simulink model "SMDFR"  (R2024b)
settings: Solver=ode15s  StartTime=1  StopTime=1200  FixedStep=0.01  RelTol=1e-3
model workspace (MAT data in the model file):
  ACS_lambda = 0.000161129786201
  A_cucl = 134.446
  A_cucl2 = 134.446
  A_cuocl = 213.991
  A_d = 217.647058824
  A_fw = [13.6 90 13.6]
  A_h = 217.647058824
  A_h2 = 217.647058824
  A_h20 = 18.015
  A_hcl = 36.458
  A_o = 32
  A_sg = 370
  A_wc = [10.9 103 10.9]
  C_c = 140.2
  C_cucl = 0.71
  C_cuocl = 1
  C_dst = 1996000
  C_h20 = 4.48
  C_hcl = 0.8
  C_hst = 1996000
  C_i0 = [429000000000000; 4.15e+15; 3.83e+15; 1.16e+16; 5.7e+15; 1.53e+15]
  C_o = 0.918
  Ce_i0 = [701000000000000; 5.88e+15; 3.36e+15; 5.09e+15; 820000000000000; 39600000000000]
  Cr = 0.00113148387097
  Cr_m = 8.769
  Cr_m_red = 4.3845
  Cr_red = 0.000565741935484
  D = 0.16
  DPB_lambda = 0.01
  EPB_lambda = 0.01
  E_d = 5
  E_e = 5
  E_h = 5
  E_hte = 5
  G_cucl = 44.778
  G_cucl2 = 44.778
  G_cuocl = 35.6355
  G_h2 = 32
  G_h20 = 10
  G_h20i = 10
  G_h20o = 7
  G_hcl = 12.1426
  G_o = 2.66
  G_s = 27000
  H_valve = 1
  Heat = [18744000 5970000 16956000]
  IPB_lambda = 0.01
  K_d = 500
  K_h = 500
  L = 6
  LOCA1 = 0
  LOCA2 = 0
  LOCA3 = 0
  LOCA4 = 0
  LOCA_p = 0.000161129786201
  LOCA_time = 300
  LOCA_times = [408 453 64 457 317 49 140 274 479 483 79 486 ... (4000 elements, 1000x4)]
  LOPC = 0
  LOPC_p = 0.1
  LOPC_times = [214 478 363 291 271 353 3 392 464 5 413 384 ... (1000 elements, 1000x1)]
  L_ACS = 0.01
  Lambda = 1.05e-06
  M_c = [219.9 7705 219.9]
  M_cucl0 = 44.778
  M_cucl20 = 44.778
  M_f = [307.7 1164 307.7]
  M_h20 = 8
  M_hcl0 = 12.1426
  M_w = [39.3 311 39.3]
  N = 1000
  N_0 = 15000000000000
  Nodes = 3
  P_0 = 100000000
  P_decomposition = 160
  P_hydro = 167
  Pb_acs : object (value not decoded)
  Pb_pipes : object (value not decoded)
  Pi_0 = [0.158 0.6899 0.152]
  Power_lambda = 0.01
  RPB_lambda = 0.01
  T_fw = 300
  T_hpi = 100
  T_st = 900
  Tbar_c0 = 1060
  Tbar_f0 = 1288
  Tc_in = 973
  Tin_c = 973
  Tin_f = 1300
  Tout_c = 1100
  Tout_f = 1300
  V_c = 160
  V_d = 160
  V_dst = 100
  V_h = 160
  V_h2 = 160
  V_hst = 100
  V_s = 100
  V_sg = 100
  age = 0
  ages = [0 50]
  alfa_c = -8.28e-06
  alfa_f = -0.000208
  alpha = 0.9926
  alpha_1 = 1
  alpha_2 = 1
  alpha_3 = 1
  alpha_4 = 1
  beta = 0.00302
  beta_i = [7.91e-05 0.000703 0.000504 0.00117 0.000457 0.00011]
  c_pc = [140.2 140.2 140.2]
  c_pf = [400 400 400]
  c_pw = [690 690 690]
  coolpipes = [2166 2166 0]
  d_c = 10187.40024
  d_dst = 3.14
  d_hst = 3.14
  d_st = 6.123
  diesel_lambda = 0.01
  eta = 0.4
  fail_threshold = 1244
  file = 'SMDFR_Parameters'
  fuelpipes = 1027
  h_dpo = 6801000
  h_fw = [6546 4305.1 7629.5]
  h_fw_st = 4386450
  h_hpo = 7159680
  h_in = 7000
  h_out = 1000
  h_st_in = 4386450
  h_wc = [27405.4 13833.4 32177.3]
  i = 1
  j = 1
  k_d = 2.7187
  k_e = 2.7187
  k_h = 0.005
  k_hte = 2.7187
  k_sg = 500
  lambda_c = 0.184
  lambda_e = 0.1
  lambda_i = [0.0127 0.03 0.11 0.319 1.18 7.02]
  leakage = 6.5
  mdot_c = [5550.5 5550.5 5550.5]
  mdot_c_value = 5550.5
  mdot_f = [327.7 327.7 327.7]
  mdot_f_value = 327.7
  model = 'SMDFR'
  mu = 50.9722799688
  mu_f = -20.9722799688
  mu_o = 30
  n = 0.45
  nsim = 1
  p_h20 = 40
  phi_tot = 3.61e+21
  rho = 7750
  rho_0 = 0.00111
  rhoex_value = 0
  sigma = 625
  sigma_c = 5
  sigma_f = 5.83095189485
  sigma_o = 3
  step = 0.1
  t = 0.008
  tau_c = 5.43
  tau_e = 10
  tsim = 500
  v_rec = 4.16e-09
values from neighbouring files (symbols this model uses):
  ACS1_flow = 25    [Simulation_model.m]
  ACS1_response_time = randi(t_max_r_ACS-t_min_r_ACS)+t_min_r_ACS    [Failure_model.m]    (also in Failure_model_outputs.mat = 38)
  ACS2_flow = 25    [Simulation_model.m]
  ACS2_response_time = randi(t_max_r_ACS-t_min_r_ACS)+t_min_r_ACS    [Failure_model.m]    (also in Failure_model_outputs.mat = 82)
  ACS3_flow = 25    [Simulation_model.m]
  ACS3_response_time = randi(t_max_r_ACS-t_min_r_ACS)+t_min_r_ACS    [Failure_model.m]    (also in Failure_model_outputs.mat = 78)
  ACS4_flow = 25    [Simulation_model.m]
  ACS4_response_time = randi(t_max_r_ACS-t_min_r_ACS)+t_min_r_ACS    [Failure_model.m]    (also in Failure_model_outputs.mat = 42)
  ACS_1 = 1065    [Failure_model_outputs.mat]    (also in Failure_sim.m = 1200; Failure_sim_HTE_model.m = 1200)
  ACS_2 = 740    [Failure_model_outputs.mat]    (also in Failure_sim.m = 1200; Failure_sim_HTE_model.m = 1200)
  ACS_3 = 745    [Failure_model_outputs.mat]    (also in Failure_sim.m = 1200; Failure_sim_HTE_model.m = 1200)
  ACS_4 = 1055    [Failure_model_outputs.mat]    (also in Failure_sim.m = 1200; Failure_sim_HTE_model.m = 1200)
  All_Outputs = 0    [Simulation_model.m]
  EDG1_response_time = randi(t_max_r_EDG-t_min_r_EDG)+t_min_r_EDG    [Failure_model.m]    (also in Failure_model_outputs.mat = 40)
  EDG2_response_time = randi(t_max_r_EDG-t_min_r_EDG)+t_min_r_EDG    [Failure_model.m]    (also in Failure_model_outputs.mat = 125)
  EDG_1 = 203    [Failure_model_outputs.mat]
  EDG_2 = 296    [Failure_model_outputs.mat]
  LOCA1_time = 1200    [Failure_model_outputs.mat]    (also in Failure_sim.m; Failure_sim_HTE_model.m)
  LOCA2_time = 2    [Failure_model_outputs.mat]    (also in Failure_sim.m = 1200; Failure_sim_HTE_model.m = 1200)
  LOCA3_time = 1200    [Failure_model_outputs.mat]    (also in Failure_sim.m; Failure_sim_HTE_model.m)
  LOCA4_time = 4    [Failure_model_outputs.mat]    (also in Failure_sim.m = 1200; Failure_sim_HTE_model.m = 1200)
  MSLB1 = 1200    [Failure_model_outputs.mat]    (also in Failure_sim.m = fix(randsample(x_loca, 1, true, lognorm_pdf)); Failure_sim_HTE_model.m = fix(randsample(x_loca, 1, true, lognorm_pdf)))
  MSLB2 = 1200    [Failure_model_outputs.mat]    (also in Failure_sim.m = fix(randsample(x_loca, 1, true, lognorm_pdf)); Failure_sim_HTE_model.m = fix(randsample(x_loca, 1, true, lognorm_pdf)))
  MSLB3 = 1200    [Failure_model_outputs.mat]    (also in Failure_sim.m = fix(randsample(x_loca, 1, true, lognorm_pdf)); Failure_sim_HTE_model.m = fix(randsample(x_loca, 1, true, lognorm_pdf)))
  MSLB4 = 1200    [Failure_model_outputs.mat]    (also in Failure_sim.m = fix(randsample(x_loca, 1, true, lognorm_pdf)); Failure_sim_HTE_model.m = fix(randsample(x_loca, 1, true, lognorm_pdf)))
  PDP11 = 1200    [Failure_model_outputs.mat]    (also in Failure_sim.m = t_min_EDG+randi(t_max_EDG-t_min_EDG); Failure_sim_HTE_model.m = t_min_EDG+randi(t_max_EDG-t_min_EDG))
  PDP11_response_time = randi(t_max_r_EDG-t_min_r_EDG)+t_min_r_EDG    [Failure_model.m]    (also in Failure_model_outputs.mat = 78)
  PDP12 = 1200    [Failure_model_outputs.mat]    (also in Failure_sim.m = t_min_EDG+randi(t_max_EDG-t_min_EDG); Failure_sim_HTE_model.m = t_min_EDG+randi(t_max_EDG-t_min_EDG))
  PDP12_response_time = randi(t_max_r_EDG-t_min_r_EDG)+t_min_r_EDG    [Failure_model.m]    (also in Failure_model_outputs.mat = 170)
  PDP21 = 1200    [Failure_model_outputs.mat]    (also in Failure_sim.m = t_min_EDG+randi(t_max_EDG-t_min_EDG); Failure_sim_HTE_model.m = t_min_EDG+randi(t_max_EDG-t_min_EDG))
  PDP21_response_time = randi(t_max_r_EDG-t_min_r_EDG)+t_min_r_EDG    [Failure_model.m]    (also in Failure_model_outputs.mat = 91)
  PDP22 = 1200    [Failure_model_outputs.mat]    (also in Failure_sim.m = t_min_EDG+randi(t_max_EDG-t_min_EDG); Failure_sim_HTE_model.m = t_min_EDG+randi(t_max_EDG-t_min_EDG))
  PDP22_response_time = randi(t_max_r_EDG-t_min_r_EDG)+t_min_r_EDG    [Failure_model.m]    (also in Failure_model_outputs.mat = 79)
  PDP31 = 1200    [Failure_model_outputs.mat]    (also in Failure_sim.m = t_min_EDG+randi(t_max_EDG-t_min_EDG); Failure_sim_HTE_model.m = t_min_EDG+randi(t_max_EDG-t_min_EDG))
  PDP31_response_time = randi(t_max_r_EDG-t_min_r_EDG)+t_min_r_EDG    [Failure_model.m]    (also in Failure_model_outputs.mat = 43)
  PDP32 = 1200    [Failure_model_outputs.mat]    (also in Failure_sim.m = t_min_EDG+randi(t_max_EDG-t_min_EDG); Failure_sim_HTE_model.m = t_min_EDG+randi(t_max_EDG-t_min_EDG))
  PDP32_response_time = randi(t_max_r_EDG-t_min_r_EDG)+t_min_r_EDG    [Failure_model.m]    (also in Failure_model_outputs.mat = 68)
  PDP41 = 1200    [Failure_model_outputs.mat]    (also in Failure_sim.m = t_min_EDG+randi(t_max_EDG-t_min_EDG); Failure_sim_HTE_model.m = t_min_EDG+randi(t_max_EDG-t_min_EDG))
  PDP41_response_time = randi(t_max_r_EDG-t_min_r_EDG)+t_min_r_EDG    [Failure_model.m]    (also in Failure_model_outputs.mat = 85)
  PDP42 = 1200    [Failure_model_outputs.mat]    (also in Failure_sim.m = t_min_EDG+randi(t_max_EDG-t_min_EDG); Failure_sim_HTE_model.m = t_min_EDG+randi(t_max_EDG-t_min_EDG))
  PDP42_response_time = randi(t_max_r_EDG-t_min_r_EDG)+t_min_r_EDG    [Failure_model.m]    (also in Failure_model_outputs.mat = 34)
  Power = 1200    [Failure_model_outputs.mat]    (also in Failure_sim.m = fix(randsample(x_loca, 1, true, lognorm_pdf)); Failure_sim_HTE_model.m = fix(randsample(x_loca, 1, true, lognorm_pdf)))
libraries: SMDFR_lib x8
settings Model: Creator=leona  LastModifiedBy=stefanomarchetti
settings OptimizationCC: ReuseModelBlockBuffer=off
settings DebuggingCC: UnconnectedInputMsg=warning  UnconnectedOutputMsg=warning  UnconnectedLineMsg=warning
settings ModelReferenceCC: EnableRefExpFcnMdlSchedulingChecks=on
settings RTWCC: GPUComputeCapability=3.5  DLArmComputeVersion=19.05

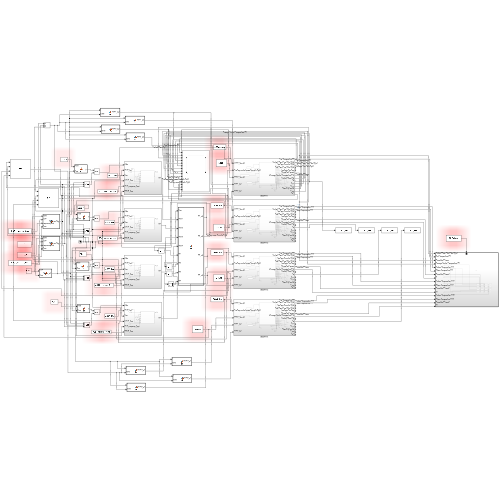
[thumbnail: Simulink's stored preview of the top-level diagram]
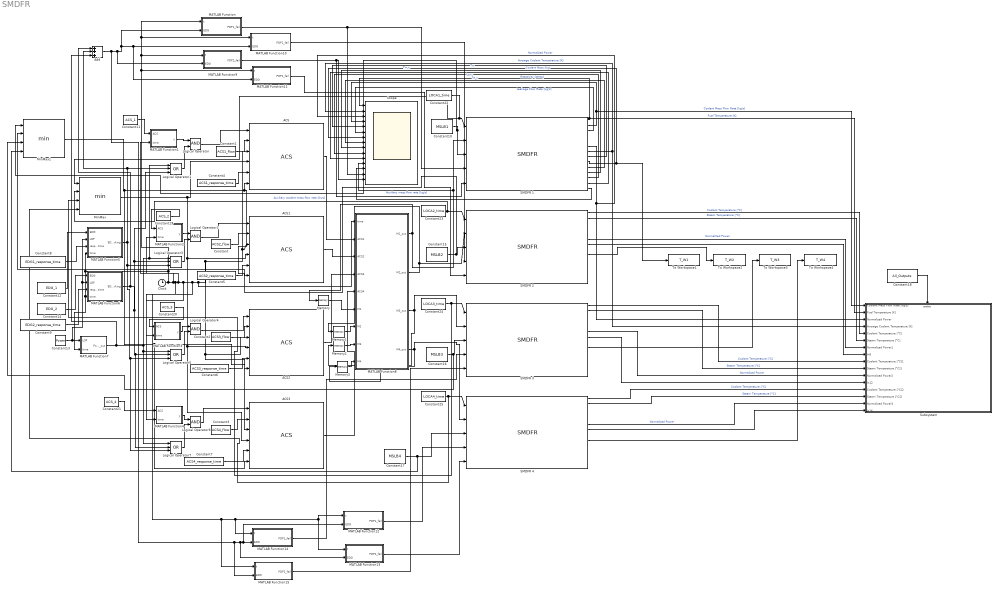
== system SMDFR ==
  ACS{,1..3} (4 alike) : SMDFR_lib/ACS  SystemSampleTime=-1  VariantActivationTime=update diagram  AllowFlexibleInterface=on  Latency=0  AutoFrameSizeCalculation=off
  Add : Sum  Inputs=+++
  Clock : Clock
  Constant : Constant  Value=ACS2_flow
  Constant1 : Constant  Value=ACS1_flow
  Constant10 : Constant  Value=MSLB1
  Constant11 : Constant  Value=ACS_1
  Constant12 : Constant  Value=EDG_1
  Constant13 : Constant  Value=Power
  Constant14 : Constant  Value=EDG_2
  Constant15 : Constant  Value=MSLB2
  Constant16 : Constant  Value=MSLB3
  Constant17 : Constant  Value=MSLB4
  Constant18 : Constant  Value=All_Outputs
  Constant19 : Constant  Value=ACS_2
  Constant2 : Constant  Value=ACS3_flow
  Constant20 : Constant  Value=ACS_3
  Constant21 : Constant  Value=ACS_4
  Constant22 : Constant  Value=LOCA1_time
  Constant23 : Constant  Value=LOCA2_time
  Constant24 : Constant  Value=LOCA3_time
  Constant25 : Constant  Value=LOCA4_time
  Constant3 : Constant  Value=ACS4_flow
  Constant4 : Constant  Value=ACS1_response_time
  Constant5 : Constant  Value=ACS2_response_time
  Constant6 : Constant  Value=ACS3_response_time
  Constant7 : Constant  Value=ACS4_response_time
  Constant8 : Constant  Value=EDG1_response_time
  Constant9 : Constant  Value=EDG2_response_time
  Logical Operator{,2,4,6} (4 alike) : Logic  AllPortsSameDT=off  OutDataTypeStr=boolean
  Logical Operator{1,3,5,7} (4 alike) : Logic  Operator=OR  Inputs=3  AllPortsSameDT=off  OutDataTypeStr=boolean
  MATLAB Function : MATLAB Function  TreatAsAtomicUnit=on
  MATLAB Function1 : MATLAB Function  TreatAsAtomicUnit=on
  MATLAB Function10 : MATLAB Function  TreatAsAtomicUnit=on
  MATLAB Function11 : MATLAB Function  TreatAsAtomicUnit=on
  MATLAB Function12 : MATLAB Function  TreatAsAtomicUnit=on
  MATLAB Function13 : MATLAB Function  TreatAsAtomicUnit=on
  MATLAB Function14 : MATLAB Function  TreatAsAtomicUnit=on
  MATLAB Function15 : MATLAB Function  TreatAsAtomicUnit=on
  MATLAB Function2 : MATLAB Function  TreatAsAtomicUnit=on
  MATLAB Function3 : MATLAB Function  TreatAsAtomicUnit=on
  MATLAB Function4 : MATLAB Function  TreatAsAtomicUnit=on
  MATLAB Function5 : MATLAB Function  TreatAsAtomicUnit=on
  MATLAB Function6 : MATLAB Function  TreatAsAtomicUnit=on
  MATLAB Function7 : MATLAB Function  TreatAsAtomicUnit=on
  MATLAB Function8 : MATLAB Function  TreatAsAtomicUnit=on
  MATLAB Function9 : MATLAB Function  TreatAsAtomicUnit=on
  Memory{,1..3} (4 alike) : Memory
  MinMax : MinMax  Inputs=4
  MinMax1 : MinMax  Inputs=4
  SMDFR 1 : SMDFR_lib/SMDFR  SystemSampleTime=-1  VariantActivationTime=update diagram  AllowFlexibleInterface=on  Latency=0  AutoFrameSizeCalculation=off
  SMDFR 2 : SMDFR_lib/SMDFR  SystemSampleTime=-1  VariantActivationTime=update diagram  AllowFlexibleInterface=on  Latency=0  AutoFrameSizeCalculation=off
      link override SMDFR/SMDFR 1/Constant10: Value=mdot_c_faultcase_2
  SMDFR 3 : SMDFR_lib/SMDFR  SystemSampleTime=-1  VariantActivationTime=update diagram  AllowFlexibleInterface=on  Latency=0  AutoFrameSizeCalculation=off
      link override SMDFR/SMDFR 1/Constant10: Value=mdot_c_faultcase_3
  SMDFR 4 : SMDFR_lib/SMDFR  SystemSampleTime=-1  VariantActivationTime=update diagram  AllowFlexibleInterface=on  Latency=0  AutoFrameSizeCalculation=off
      link override SMDFR/SMDFR 1/Constant10: Value=mdot_c_faultcase_3
  Scope : Scope  NumInputPorts=15
  Subsystem : Subsystem
  To Workspace1 : ToWorkspace  VariableName=T_W1  SampleTime=1
  To Workspace2 : ToWorkspace  VariableName=T_W2  SampleTime=1
  To Workspace3 : ToWorkspace  VariableName=T_W3  SampleTime=1
  To Workspace4 : ToWorkspace  VariableName=T_W4  SampleTime=1
  wires:
  SMDFR 1/1 -> Subsystem/2(Fuel Temperature [K]), Scope/1  "Fuel Temperature [K]"
  SMDFR 1/2 -> Subsystem/1(Coolant Mass Flow Rate [kg/s]), Scope/4  "Coolant Mass Flow Rate [kg/s]"
  SMDFR 1/6 -> Subsystem/3(Normalized Power), Scope/3  "Normalized Power"
  ACS/1 -> MATLAB Function8/2(ACS1)  "Auxiliary coolant mass flow rate [ks/s]"
  ACS1/1 -> MATLAB Function8/3(ACS2)
  ACS2/1 -> MATLAB Function8/4(ACS3)
  ACS3/1 -> MATLAB Function8/5(ACS4)
  MATLAB Function5/1(EDG_working) -> Logical Operator1/2, Add/2, Logical Operator7/3, Logical Operator5/3, Logical Operator3/3
  Logical Operator1/1 -> Logical Operator/2
  Logical Operator/1 -> ACS/1
  Logical Operator3/1 -> Logical Operator2/2
  MATLAB Function7/1(Power_out) -> Add/3, Logical Operator1/1, Logical Operator3/1, Logical Operator7/1, Logical Operator5/1
  MATLAB Function6/1(EDG_working) -> Add/1, Logical Operator7/2, Logical Operator5/2, Logical Operator1/3, Logical Operator3/2
  Logical Operator2/1 -> ACS1/1
  Logical Operator5/1 -> Logical Operator4/2
  Logical Operator4/1 -> ACS2/1
  Logical Operator7/1 -> Logical Operator6/2
  Logical Operator6/1 -> ACS3/1
  Clock/1 -> MATLAB Function11/1(t), MATLAB Function10/1(t), MATLAB Function/1(t), MATLAB Function9/1(t), MATLAB Function6/4(time), MATLAB Function7/2(time), MATLAB Function5/4(time), MATLAB Function2/2(time), MATLAB Function15/1(t), MATLAB Function14/1(t), MATLAB Function13/1(t), MATLAB Function12/1(t), MATLAB Function1/2(time), MATLAB Function3/2(time), MATLAB Function4/2(time), MATLAB Function8/1(time), ACS1/3, ACS/3, ACS3/3, ACS2/3
  Constant/1 -> ACS1/2
  Constant1/1 -> ACS/2
  Constant2/1 -> ACS2/2
  Constant3/1 -> ACS3/2
  Constant11/1 -> MATLAB Function1/1(ACS)
  Constant19/1 -> MATLAB Function2/1(ACS)
  Constant20/1 -> MATLAB Function3/1(ACS)
  Constant21/1 -> MATLAB Function4/1(ACS)
  Constant22/1 -> MinMax/1, SMDFR 1/1
  Constant23/1 -> SMDFR 2/1, MinMax/2
  Constant24/1 -> MinMax/3, SMDFR 3/1
  Constant25/1 -> SMDFR 4/1, MinMax/4
  MATLAB Function1/1(y) -> Logical Operator/1
  MATLAB Function2/1(y) -> Logical Operator2/1
  MATLAB Function3/1(y) -> Logical Operator4/1
  MATLAB Function4/1(y) -> Logical Operator6/1
  Constant12/1 -> MATLAB Function5/1(EDG)
  Constant14/1 -> MATLAB Function6/1(EDG)
  Constant13/1 -> MATLAB Function5/2(LOP), MATLAB Function6/2(LOP), MATLAB Function7/1(LOP)
  MATLAB Function8/1(M1_out) -> Memory/1, SMDFR 1/2, Scope/12  "Auxiliary mass flow rate [kg/s]"
  MATLAB Function8/2(M2_out) -> Memory1/1, SMDFR 2/2
  MATLAB Function8/3(M3_out) -> SMDFR 3/2, Memory2/1
  MATLAB Function8/4(M4_out) -> SMDFR 4/2, Memory3/1
  MinMax/1 -> ACS/4, ACS1/4, ACS3/4, ACS2/4
  Constant8/1 -> MATLAB Function5/3(response_time)
  Constant9/1 -> MATLAB Function6/3(response_time)
  Constant4/1 -> ACS/5
  Constant5/1 -> ACS1/5
  Constant6/1 -> ACS2/5
  Constant7/1 -> ACS3/5
  Memory/1 -> MATLAB Function8/6(M1)
  Memory1/1 -> MATLAB Function8/7(M2)
  Memory2/1 -> MATLAB Function8/8(M3)
  Memory3/1 -> MATLAB Function8/9(M4)
  SMDFR 1/7 -> Subsystem/4(Average Coolant Temperature [K]), Scope/2  "Average Coolant Temperature [K]"
  SMDFR 1/8 -> Scope/5  "Coolant Mass [kg]"
  SMDFR 1/3 -> Scope/6  "Leakage Flow Rate [kg/s]"
  SMDFR 1/9 -> To Workspace1/1, Scope/7  "Tw"
  SMDFR 1/10 -> Scope/8  "Te_c"
  SMDFR 1/11 -> Scope/9  "Tin_c"
  SMDFR 1/12 -> Scope/10  "Reactivity [cents]"
  SMDFR 1/13 -> Scope/11  "h_wc"
  SMDFR 2/9 -> To Workspace2/1
  SMDFR 3/9 -> To Workspace3/1
  SMDFR 4/9 -> To Workspace4/1
  SMDFR 1/14 -> Scope/13
  MATLAB Function/1(PDP1_fail) -> Scope/14, SMDFR 1/4
  Constant10/1 -> MinMax1/1, SMDFR 1/3
  Constant15/1 -> MinMax1/2, SMDFR 2/3
  Constant16/1 -> MinMax1/3, SMDFR 3/3
  Constant17/1 -> MinMax1/4, SMDFR 4/3
  MATLAB Function10/1(PDP1_fail) -> SMDFR 2/4
  MATLAB Function12/1(PDP1_fail) -> SMDFR 4/4
  MATLAB Function14/1(PDP1_fail) -> SMDFR 3/4
  Add/1 -> MATLAB Function15/2(EDG), MATLAB Function13/2(EDG), MATLAB Function12/2(EDG), MATLAB Function14/2(EDG), MATLAB Function9/2(EDG), MATLAB Function11/2(EDG), MATLAB Function10/2(EDG), MATLAB Function/2(EDG)
  MinMax1/1 -> ACS1/6, ACS/6, ACS2/6, ACS3/6
  MATLAB Function13/1(PDP2_fail) -> SMDFR 4/5
  MATLAB Function15/1(PDP2_fail) -> SMDFR 3/5
  MATLAB Function9/1(PDP2_fail) -> Scope/15, SMDFR 1/5
  MATLAB Function11/1(PDP2_fail) -> SMDFR 2/5
  SMDFR 2/1 -> Subsystem/5(Coolant Temperature [°C])  "Coolant Temperature [°C]"
  SMDFR 2/2 -> Subsystem/6(Steam Temperature [°C])  "Steam Temperature [°C]"
  SMDFR 2/6 -> Subsystem/7(Normalized Power1)  "Normalized Power"
  SMDFR 2/7 -> Subsystem/8(In8)
  SMDFR 3/1 -> Subsystem/9(Coolant Temperature [°C]1)  "Coolant Temperature [°C]"
  SMDFR 3/2 -> Subsystem/10(Steam Temperature [°C]1)  "Steam Temperature [°C]"
  SMDFR 3/6 -> Subsystem/11(Normalized Power2)  "Normalized Power"
  SMDFR 3/7 -> Subsystem/12(In12)
  SMDFR 4/1 -> Subsystem/13(Coolant Temperature [°C]2)  "Coolant Temperature [°C]"
  SMDFR 4/2 -> Subsystem/14(Steam Temperature [°C]2)  "Steam Temperature [°C]"
  SMDFR 4/6 -> Subsystem/15(Normalized Power3)  "Normalized Power"
  SMDFR 4/7 -> Subsystem/16(In16)
  Constant18/1 -> Subsystem/Enable

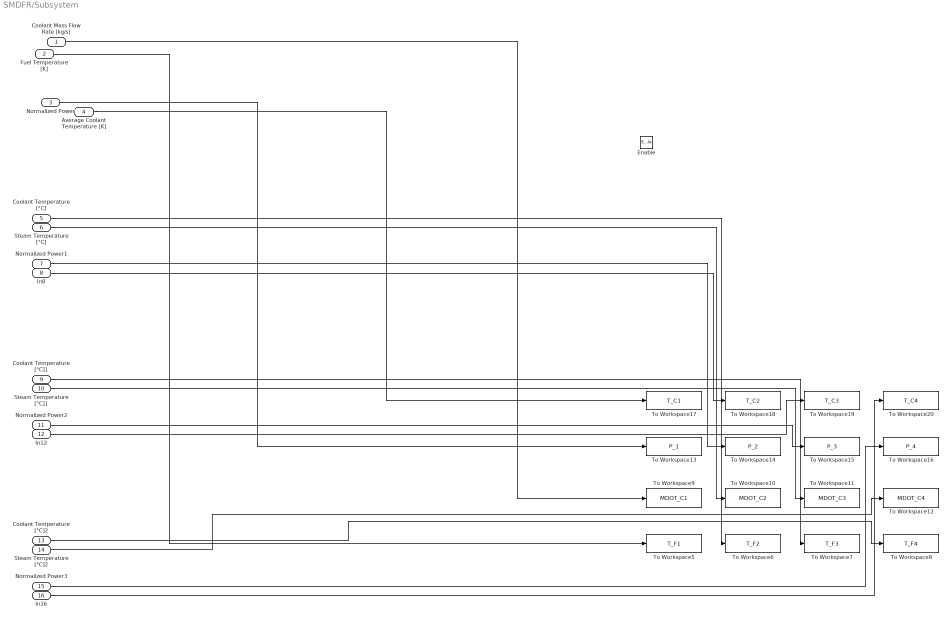
== system SMDFR/Subsystem ==
  Coolant Mass Flow Rate [kg/s] : Inport
  Fuel Temperature [K] : Inport  Port=2
  Normalized Power : Inport  Port=3
  Average Coolant Temperature [K] : Inport  Port=4
  Coolant Temperature [°C] : Inport  Port=5
  Steam Temperature [°C] : Inport  Port=6
  Normalized Power1 : Inport  Port=7
  In8 : Inport  Port=8
  Coolant Temperature [°C]1 : Inport  Port=9
  Steam Temperature [°C]1 : Inport  Port=10
  Normalized Power2 : Inport  Port=11
  In12 : Inport  Port=12
  Coolant Temperature [°C]2 : Inport  Port=13
  Steam Temperature [°C]2 : Inport  Port=14
  Normalized Power3 : Inport  Port=15
  In16 : Inport  Port=16
  Enable : EnablePort
  To Workspace10 : ToWorkspace  VariableName=MDOT_C2  SampleTime=1
  To Workspace11 : ToWorkspace  VariableName=MDOT_C3  SampleTime=1
  To Workspace12 : ToWorkspace  VariableName=MDOT_C4  SampleTime=1
  To Workspace13 : ToWorkspace  VariableName=P_1  SampleTime=1
  To Workspace14 : ToWorkspace  VariableName=P_2  SampleTime=1
  To Workspace15 : ToWorkspace  VariableName=P_3  SampleTime=1
  To Workspace16 : ToWorkspace  VariableName=P_4  SampleTime=1
  To Workspace17 : ToWorkspace  VariableName=T_C1  SampleTime=1
  To Workspace18 : ToWorkspace  VariableName=T_C2  SampleTime=1
  To Workspace19 : ToWorkspace  VariableName=T_C3  SampleTime=1
  To Workspace20 : ToWorkspace  VariableName=T_C4  SampleTime=1
  To Workspace5 : ToWorkspace  VariableName=T_F1  SampleTime=1
  To Workspace6 : ToWorkspace  VariableName=T_F2  SampleTime=1
  To Workspace7 : ToWorkspace  VariableName=T_F3  SampleTime=1
  To Workspace8 : ToWorkspace  VariableName=T_F4  SampleTime=1
  To Workspace9 : ToWorkspace  VariableName=MDOT_C1  SampleTime=1
  wires:
  Normalized Power/1 -> To Workspace13/1
  Coolant Temperature [°C]1/1 -> To Workspace7/1
  Coolant Mass Flow Rate [kg/s]/1 -> To Workspace9/1
  Average Coolant Temperature [K]/1 -> To Workspace17/1
  Fuel Temperature [K]/1 -> To Workspace5/1
  Coolant Temperature [°C]2/1 -> To Workspace8/1
  In12/1 -> To Workspace19/1
  In8/1 -> To Workspace18/1
  Coolant Temperature [°C]/1 -> To Workspace6/1
  Steam Temperature [°C]/1 -> To Workspace10/1
  In16/1 -> To Workspace20/1
  Normalized Power1/1 -> To Workspace14/1
  Steam Temperature [°C]1/1 -> To Workspace11/1
  Normalized Power2/1 -> To Workspace15/1
  Steam Temperature [°C]2/1 -> To Workspace12/1
  Normalized Power3/1 -> To Workspace16/1

== matlab function SMDFR/MATLAB Function8 ==
  data: M1_out output; time input; ACS1 input; ACS2 input; ACS3 input; ACS4 input; M2_out output; M3_out output; M4_out output; M1 input; M2 input; M3 input; M4 input; LOCA1_time parameter; LOCA2_time parameter; LOCA3_time parameter; LOCA4_time parameter; MSLB1 parameter; MSLB2 parameter; MSLB3 parameter; MSLB4 parameter
function [M1_out,M2_out,M3_out,M4_out] = fcn(time,ACS1,ACS2,ACS3,ACS4,M1,M2,M3,M4,LOCA1_time, LOCA2_time, LOCA3_time, LOCA4_time, MSLB1, MSLB2, MSLB3, MSLB4)
LOCA_fail=zeros(4,1);
increment = 0.1;
if LOCA1_time < time
    LOCA_fail(1) = 1;
end
if LOCA2_time < time
    LOCA_fail(2) = 1;
end
if LOCA3_time < time
    LOCA_fail(3) = 1;
end
if LOCA4_time < time
    LOCA_fail(4) = 1;
end

if sum(LOCA_fail)>0 && MSLB1>time && MSLB2>time && MSLB3>time && MSLB4>time
    M_out = LOCA_fail/sum(LOCA_fail)*(ACS1+ACS2+ACS3+ACS4);
    if mod(time,1)==0
        if M_out(1) > M1
            M1_out=min(M_out(1),M1+increment);
        else
            if M_out(1)<M1
                M1_out=max(M_out(1),M1-increment);
            else
                M1_out=M_out(1);
            end
        end
    else
        M1_out=M1;
    end
    if mod(time,1)==0
        if M_out(2) > M2
            M2_out=min(M_out(2),M2+increment);
        else
            if M_out(2)<M2
                M2_out=max(M_out(2),M2-increment);
            else
                M2_out=M_out(2);
            end
        end
    else
        M2_out=M2;
    end
    if mod(time,1)==0
        if M_out(3) > M3
            M3_out=min(M_out(3),M3+increment);
        else
            if M_out(3)<M3
                M3_out=max(M_out(3),M3-increment);
            else
                M3_out=M_out(3);
            end
        end
    else
        M3_out=M3;
    end
    if mod(time,1)==0
        if M_out(4) > M4
            M4_out=min(M_out(4),M4+increment);
        else
            if M_out(4)<M4
                M4_out=max(M_out(4),M4-increment);
            else
                M4_out=M_out(4);
            end
        end
    else
        M4_out=M4;
    end
else
    M_out=zeros(4,1);
    M1_out = M_out(1);
    M2_out = M_out(2);
    M3_out = M_out(3);
    M4_out = M_out(4);
end

factor=40*10;
if MSLB1<time
    M1_out = M1_out+(ACS1+ACS2+ACS3+ACS4)*factor;
end
if MSLB2<time
    M2_out = M2_out+(ACS1+ACS2+ACS3+ACS4)*factor;
end
if MSLB3<time
    M3_out = M3_out+(ACS1+ACS2+ACS3+ACS4)*factor;
end
if MSLB4<time
    M4_out = M4_out+(ACS1+ACS2+ACS3+ACS4)*factor;
end


end

== matlab function SMDFR/MATLAB Function ==
  data: t input; PDP1_fail output; MSLB1 parameter; PDP11_response_time parameter; PDP11 parameter; EDG input
function PDP1_fail = fcn(t,MSLB1, PDP11_response_time, PDP11, EDG)

if ((t<PDP11 || EDG) && t>(MSLB1+PDP11_response_time)) 
    PDP1_fail=0;
else
    PDP1_fail=1;
end

== matlab function SMDFR/MATLAB Function9 ==
  data: t input; PDP2_fail output; MSLB1 parameter; PDP12_response_time parameter; PDP12 parameter; EDG input
function PDP2_fail = fcn(t,MSLB1, PDP12_response_time, PDP12, EDG)

if ((t<PDP12 || EDG) && t>(MSLB1+PDP12_response_time)) 
    PDP2_fail=0;
else
    PDP2_fail=1;
end

== matlab function SMDFR/MATLAB Function10 ==
  data: t input; PDP1_fail output; MSLB2 parameter; PDP21_response_time parameter; PDP21 parameter; EDG input
function PDP1_fail = fcn(t,MSLB2, PDP21_response_time, PDP21, EDG)

if ((t<PDP21 || EDG) && t>(MSLB2+PDP21_response_time)) 
    PDP1_fail=0;
else
    PDP1_fail=1;
end

== matlab function SMDFR/MATLAB Function11 ==
  data: t input; PDP2_fail output; MSLB2 parameter; PDP22_response_time parameter; PDP22 parameter; EDG input
function PDP2_fail = fcn(t,MSLB2, PDP22_response_time, PDP22, EDG)

if ((t<PDP22 || EDG) && t>(MSLB2+PDP22_response_time)) 
    PDP2_fail=0;
else
    PDP2_fail=1;
end

== matlab function SMDFR/MATLAB Function12 ==
  data: t input; PDP1_fail output; MSLB4 parameter; PDP41_response_time parameter; PDP41 parameter; EDG input
function PDP1_fail = fcn(t,MSLB4, PDP41_response_time, PDP41, EDG)

if ((t<PDP41 || EDG) && t>(MSLB4+PDP41_response_time)) 
    PDP1_fail=0;
else
    PDP1_fail=1;
end

== matlab function SMDFR/MATLAB Function13 ==
  data: t input; PDP2_fail output; MSLB4 parameter; PDP42_response_time parameter; PDP42 parameter; EDG input
function PDP2_fail = fcn(t,MSLB4, PDP42_response_time, PDP42, EDG)

if ((t<PDP42 || EDG) && t>(MSLB4+PDP42_response_time)) 
    PDP2_fail=0;
else
    PDP2_fail=1;
end

== matlab function SMDFR/MATLAB Function14 ==
  data: t input; PDP1_fail output; MSLB3 parameter; PDP31_response_time parameter; PDP31 parameter; EDG input
function PDP1_fail = fcn(t,MSLB3, PDP31_response_time, PDP31, EDG)

if ((t<PDP31 || EDG) && t>(MSLB3+PDP31_response_time)) 
    PDP1_fail=0;
else
    PDP1_fail=1;
end

== matlab function SMDFR/MATLAB Function15 ==
  data: t input; PDP2_fail output; MSLB3 parameter; PDP32_response_time parameter; PDP32 parameter; EDG input
function PDP2_fail = fcn(t,MSLB3, PDP32_response_time, PDP32, EDG)

if ((t<PDP32 || EDG) && t>(MSLB3+PDP32_response_time)) 
    PDP2_fail=0;
else
    PDP2_fail=1;
end

== matlab function SMDFR/MATLAB Function2 ==
  data: ACS input; y output; time input
function y = fcn(ACS,time)

if time > ACS
    y=0;
else
    y=1;
end

== matlab function SMDFR/MATLAB Function1 ==
  data: ACS input; y output; time input
function y = fcn(ACS,time)

if time > ACS
    y=0;
else
    y=1;
end

== matlab function SMDFR/MATLAB Function3 ==
  data: ACS input; y output; time input
function y = fcn(ACS,time)

if time > ACS
    y=0;
else
    y=1;
end

== matlab function SMDFR/MATLAB Function4 ==
  data: ACS input; y output; time input
function y= fcn(ACS,time)

if time > ACS
    y=0;
else
    y=1;
end

== matlab function SMDFR/MATLAB Function5 ==
  data: EDG input; LOP input; response_time input; EDG_working output; time input
function EDG_working = fcn(EDG,LOP, response_time, time)

if time > EDG
    EDG_working=0;
else
    if (time-LOP)>response_time
        EDG_working=1;
    else
        EDG_working=0;
    end
end

== matlab function SMDFR/MATLAB Function6 ==
  data: EDG input; LOP input; response_time input; EDG_working output; time input
function EDG_working = fcn(EDG,LOP, response_time, time)

if time > EDG
    EDG_working=0;
else
    if (time-LOP)>response_time
        EDG_working=1;
    else
        EDG_working=0;
    end
end

== matlab function SMDFR/MATLAB Function7 ==
  data: LOP input; Power_out output; time input
function Power_out = fcn(LOP,time)

if time > LOP
    Power_out=0;
else
    Power_out=1;
end
